simulink library "BEML_EMU_PantographInput_Lib"  (R2019b)
settings: Solver=VariableStepAuto  StartTime=0.0  StopTime=10.0  RelTol=1e-3
undefined symbols (not defined in the file): Control, Electrical, Environment, LineVoltage, NeutralSection, OverheadLinePresent, PantoADDFault, PantoControlPower, PantoDownCommand, PantographSampleTime, PantoIsolationCommand, PantoLoweringFailure, PantoMotorPower, PantoORDFault, PantoRaiseFailure, PantoUpCommand, Pneumatics
settings Model: Creator=rleighton  LastModifiedBy=hinganes
settings DataIOCC: ReturnWorkspaceOutputs=off
settings DebuggingCC: ArithmeticOperatorsInVariantConditions=warning
settings SFSimCC: SimUseLocalCustomCode=off  CustomCodeUndefinedFunction=UseInterfaceOnly
settings RTWCC: RTWUseLocalCustomCode=off

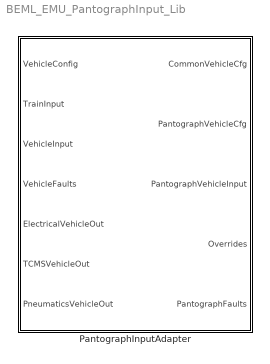
== system BEML_EMU_PantographInput_Lib ==
  PantographInputAdapter : Subsystem  TreatAsAtomicUnit=on  SystemSampleTime=PantographSampleTime

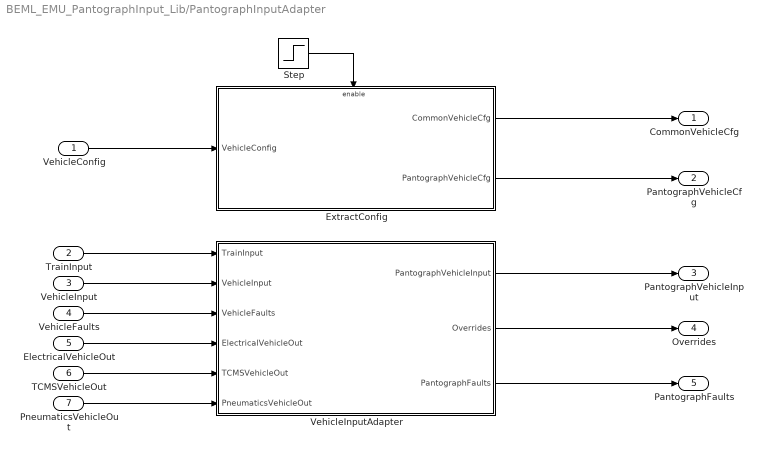
== system BEML_EMU_PantographInput_Lib/PantographInputAdapter ==
  VehicleConfig : Inport
  TrainInput : Inport  Port=2
  VehicleInput : Inport  Port=3
  VehicleFaults : Inport  Port=4
  ElectricalVehicleOut : Inport  Port=5
  TCMSVehicleOut : Inport  Port=6
  PneumaticsVehicleOut : Inport  Port=7
  ExtractConfig : Subsystem
  Step : Step  Before=1  After=0
  VehicleInputAdapter : Subsystem
  CommonVehicleCfg : Outport  VectorParamsAs1DForOutWhenUnconnected=off
  PantographVehicleCfg : Outport  Port=2  VectorParamsAs1DForOutWhenUnconnected=off
  PantographVehicleInput : Outport  Port=3  VectorParamsAs1DForOutWhenUnconnected=off
  Overrides : Outport  Port=4  VectorParamsAs1DForOutWhenUnconnected=off
  PantographFaults : Outport  Port=5  VectorParamsAs1DForOutWhenUnconnected=off
  wires:
  TrainInput/1 -> VehicleInputAdapter/1(TrainInput)
  VehicleInput/1 -> VehicleInputAdapter/2(VehicleInput)
  ElectricalVehicleOut/1 -> VehicleInputAdapter/4(ElectricalVehicleOut)
  PneumaticsVehicleOut/1 -> VehicleInputAdapter/6(PneumaticsVehicleOut)
  VehicleConfig/1 -> ExtractConfig/1(VehicleConfig)
  ExtractConfig/1(CommonVehicleCfg) -> CommonVehicleCfg/1
  ExtractConfig/2(PantographVehicleCfg) -> PantographVehicleCfg/1
  Step/1 -> ExtractConfig/Enable
  VehicleFaults/1 -> VehicleInputAdapter/3(VehicleFaults)
  VehicleInputAdapter/1(PantographVehicleInput) -> PantographVehicleInput/1
  VehicleInputAdapter/2(Overrides) -> Overrides/1
  VehicleInputAdapter/3(PantographFaults) -> PantographFaults/1
  TCMSVehicleOut/1 -> VehicleInputAdapter/5(TCMSVehicleOut)

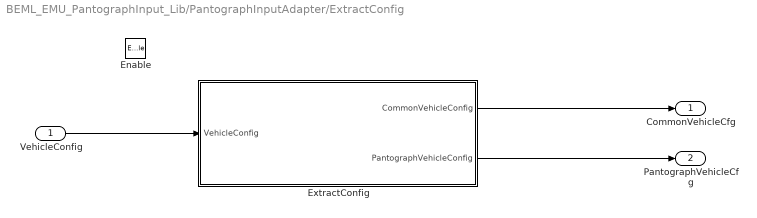
== system BEML_EMU_PantographInput_Lib/PantographInputAdapter/ExtractConfig ==
  VehicleConfig : Inport
  Enable : EnablePort
  ExtractConfig : Subsystem
  CommonVehicleCfg : Outport  VectorParamsAs1DForOutWhenUnconnected=off
  PantographVehicleCfg : Outport  Port=2  VectorParamsAs1DForOutWhenUnconnected=off
  wires:
  ExtractConfig/2(PantographVehicleConfig) -> PantographVehicleCfg/1
  ExtractConfig/1(CommonVehicleConfig) -> CommonVehicleCfg/1
  VehicleConfig/1 -> ExtractConfig/1(VehicleConfig)

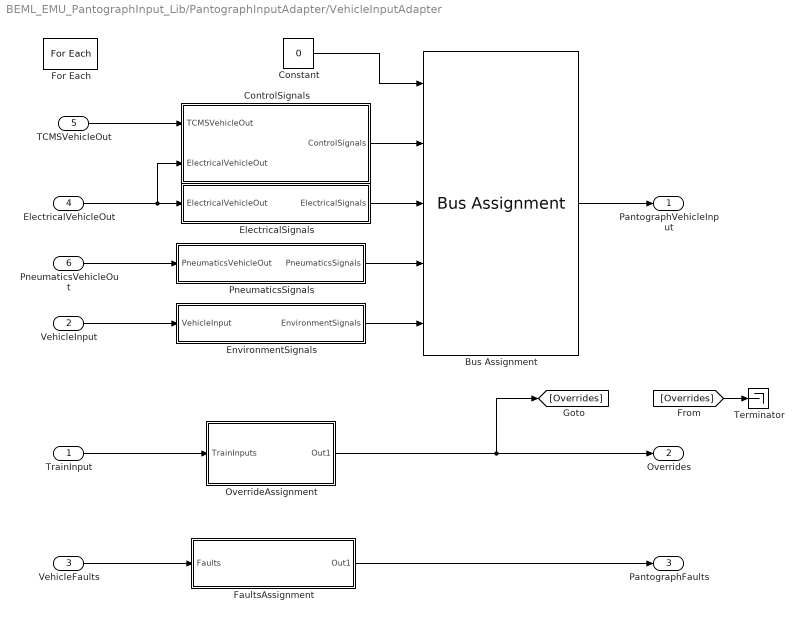
== system BEML_EMU_PantographInput_Lib/PantographInputAdapter/VehicleInputAdapter ==
  TrainInput : Inport
  VehicleInput : Inport  Port=2  Partition=on  PartitionDimension=1  PartitionWidth=1  PartitionOffset=0
  VehicleFaults : Inport  Port=3  Partition=on  PartitionDimension=1  PartitionWidth=1  PartitionOffset=0
  ElectricalVehicleOut : Inport  Port=4  Partition=on  PartitionDimension=1  PartitionWidth=1  PartitionOffset=0
  TCMSVehicleOut : Inport  Port=5  Partition=on  PartitionDimension=1  PartitionWidth=1  PartitionOffset=0
  PneumaticsVehicleOut : Inport  Port=6  Partition=on  PartitionDimension=1  PartitionWidth=1  PartitionOffset=0
  Bus Assignment : BusAssignment  AssignedSignals=Control,Electrical,Pneumatics,Environment
  Constant : Constant  Value=0  OutDataTypeStr=Bus: BD_PantographSystem_In_Vehicle
  ControlSignals : Subsystem
  ElectricalSignals : Subsystem
  EnvironmentSignals : Subsystem
  FaultsAssignment : Subsystem
  For Each : ForEach  DisableCoverage=on
  OverrideAssignment : Subsystem
  PneumaticsSignals : Subsystem
  Terminator : Terminator
  PantographVehicleInput : Outport  ConcatenationDimension=1  VectorParamsAs1DForOutWhenUnconnected=off
  Overrides : Outport  Port=2  ConcatenationDimension=1  VectorParamsAs1DForOutWhenUnconnected=off
  PantographFaults : Outport  Port=3  ConcatenationDimension=1  VectorParamsAs1DForOutWhenUnconnected=off
  wires:
  FaultsAssignment/1(Out1) -> PantographFaults/1
  VehicleFaults/1 -> FaultsAssignment/1(Faults)
  [Overrides] -> Terminator/1
  OverrideAssignment/1(Out1) -> [Overrides], Overrides/1
  TrainInput/1 -> OverrideAssignment/1(TrainInputs)
  EnvironmentSignals/1(EnvironmentSignals) -> Bus Assignment/5
  PneumaticsSignals/1(PneumaticsSignals) -> Bus Assignment/4
  VehicleInput/1 -> EnvironmentSignals/1(VehicleInput)
  ElectricalVehicleOut/1 -> ElectricalSignals/1(ElectricalVehicleOut), ControlSignals/2(ElectricalVehicleOut)
  Constant/1 -> Bus Assignment/1
  Bus Assignment/1 -> PantographVehicleInput/1
  ElectricalSignals/1(ElectricalSignals) -> Bus Assignment/3
  ControlSignals/1(ControlSignals) -> Bus Assignment/2
  PneumaticsVehicleOut/1 -> PneumaticsSignals/1(PneumaticsVehicleOut)
  TCMSVehicleOut/1 -> ControlSignals/1(TCMSVehicleOut)

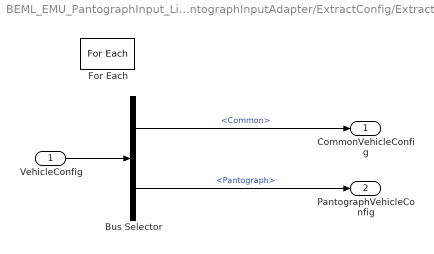
== system BEML_EMU_PantographInput_Lib/PantographInputAdapter/ExtractConfig/ExtractConfig ==
  VehicleConfig : Inport  Partition=on  PartitionDimension=1  PartitionWidth=1  PartitionOffset=0  BusOutputAsStruct=on
  Bus Selector : BusSelector  OutputSignals=Common,Pantograph
  For Each : ForEach  DisableCoverage=on
  CommonVehicleConfig : Outport  ConcatenationDimension=1  VectorParamsAs1DForOutWhenUnconnected=off
  PantographVehicleConfig : Outport  Port=2  ConcatenationDimension=1  VectorParamsAs1DForOutWhenUnconnected=off
  wires:
  VehicleConfig/1 -> Bus Selector/1
  Bus Selector/1 -> CommonVehicleConfig/1  "<Common>"
  Bus Selector/2 -> PantographVehicleConfig/1  "<Pantograph>"

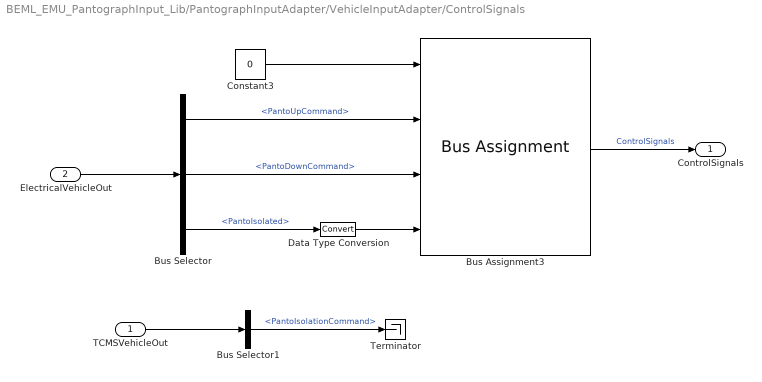
== system BEML_EMU_PantographInput_Lib/PantographInputAdapter/VehicleInputAdapter/ControlSignals ==
  TCMSVehicleOut : Inport
  ElectricalVehicleOut : Inport  Port=2
  Bus Assignment3 : BusAssignment  AssignedSignals=PantoUpCommand,PantoDownCommand,PantoIsolationCommand
  Bus Selector : BusSelector  OutputSignals=Pantograph.PantoUpCommand,Pantograph.PantoDownCommand,TCMS.PantoIsolated
  Bus Selector1 : BusSelector  OutputSignals=Control.PantographSystem.PantoIsolationCommand
  Constant3 : Constant  Value=0  OutDataTypeStr=Bus: BD_PantographSystem_In_Vehicle_Control
  Data Type Conversion : DataTypeConversion
  Terminator : Terminator
  ControlSignals : Outport
  wires:
  Data Type Conversion/1 -> Bus Assignment3/4
  Bus Selector/3 -> Data Type Conversion/1  "<PantoIsolated>"
  Bus Selector/2 -> Bus Assignment3/3  "<PantoDownCommand>"
  TCMSVehicleOut/1 -> Bus Selector1/1
  Bus Selector1/1 -> Terminator/1  "<PantoIsolationCommand>"
  ElectricalVehicleOut/1 -> Bus Selector/1
  Bus Assignment3/1 -> ControlSignals/1  "ControlSignals"
  Constant3/1 -> Bus Assignment3/1
  Bus Selector/1 -> Bus Assignment3/2  "<PantoUpCommand>"

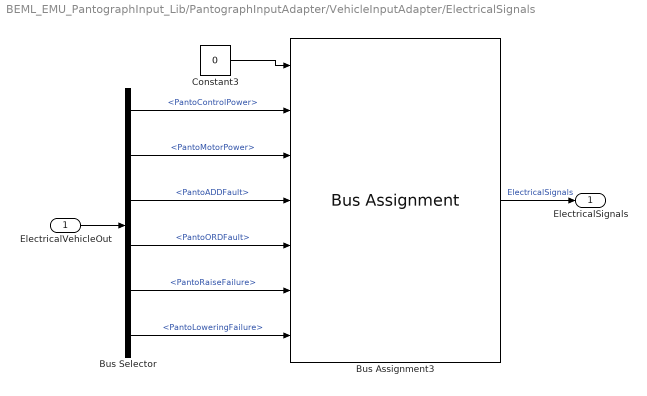
== system BEML_EMU_PantographInput_Lib/PantographInputAdapter/VehicleInputAdapter/ElectricalSignals ==
  ElectricalVehicleOut : Inport
  Bus Assignment3 : BusAssignment  AssignedSignals=PantoControlPower,PantoMotorPower,PantoADDFault,PantoORDFault,PantoRaiseFailure,PantoLoweringFailure
  Bus Selector : BusSelector  OutputSignals=Pantograph.PantoControlPower,Pantograph.PantoMotorPower,Pantograph.PantoADDFault,Pantograph.PantoORDFault,Pantograph.PantoRaiseFailure,Pantograph.PantoLoweringFailure
  Constant3 : Constant  Value=0  OutDataTypeStr=Bus: BD_PantographSystem_In_Vehicle_Electrical
  ElectricalSignals : Outport
  wires:
  Bus Selector/6 -> Bus Assignment3/7  "<PantoLoweringFailure>"
  Bus Selector/5 -> Bus Assignment3/6  "<PantoRaiseFailure>"
  Bus Selector/4 -> Bus Assignment3/5  "<PantoORDFault>"
  Bus Selector/3 -> Bus Assignment3/4  "<PantoADDFault>"
  ElectricalVehicleOut/1 -> Bus Selector/1
  Bus Assignment3/1 -> ElectricalSignals/1  "ElectricalSignals"
  Constant3/1 -> Bus Assignment3/1
  Bus Selector/1 -> Bus Assignment3/2  "<PantoControlPower>"
  Bus Selector/2 -> Bus Assignment3/3  "<PantoMotorPower>"

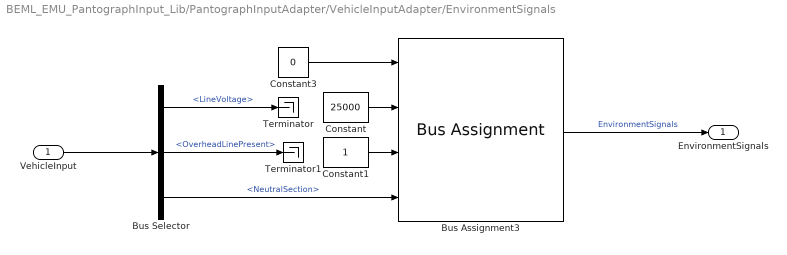
== system BEML_EMU_PantographInput_Lib/PantographInputAdapter/VehicleInputAdapter/EnvironmentSignals ==
  VehicleInput : Inport
  Bus Assignment3 : BusAssignment  AssignedSignals=LineVoltage,OverheadLinePresent,NeutralSection
  Bus Selector : BusSelector  OutputSignals=Environment.LineVoltage,Environment.OverheadLinePresent,Environment.NeutralSection
  Constant : Constant  Value=25000
  Constant1 : Constant
  Constant3 : Constant  Value=0  OutDataTypeStr=Bus: BD_PantographSystem_In_Vehicle_Environment
  Terminator : Terminator
  Terminator1 : Terminator
  EnvironmentSignals : Outport
  wires:
  Constant/1 -> Bus Assignment3/2
  Constant1/1 -> Bus Assignment3/3
  Bus Selector/3 -> Bus Assignment3/4  "<NeutralSection>"
  Bus Selector/2 -> Terminator1/1  "<OverheadLinePresent>"
  Bus Selector/1 -> Terminator/1  "<LineVoltage>"
  VehicleInput/1 -> Bus Selector/1
  Bus Assignment3/1 -> EnvironmentSignals/1  "EnvironmentSignals"
  Constant3/1 -> Bus Assignment3/1

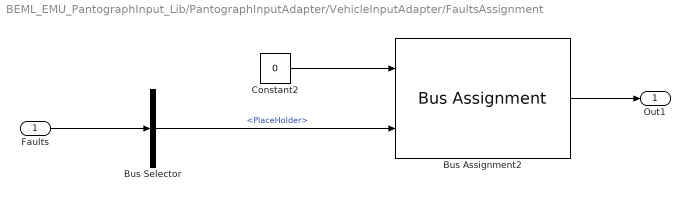
== system BEML_EMU_PantographInput_Lib/PantographInputAdapter/VehicleInputAdapter/FaultsAssignment ==
  Faults : Inport
  Bus Assignment2 : BusAssignment  AssignedSignals=PlaceHolder
  Bus Selector : BusSelector  OutputSignals=PantographFaults.PlaceHolder
  Constant2 : Constant  Value=0  OutDataTypeStr=Bus: BD_PantographSystem_In_Vehicle_Faults
  Out1 : Outport
  wires:
  Constant2/1 -> Bus Assignment2/1
  Bus Assignment2/1 -> Out1/1
  Faults/1 -> Bus Selector/1
  Bus Selector/1 -> Bus Assignment2/2  "<PlaceHolder>"

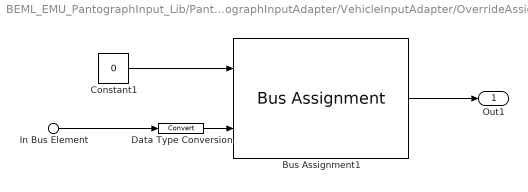
== system BEML_EMU_PantographInput_Lib/PantographInputAdapter/VehicleInputAdapter/OverrideAssignment ==
  In Bus Element : Inport  PortName=TrainInputs  Element=Overrides.AutoPowerOn
  Bus Assignment1 : BusAssignment  AssignedSignals=PantoUPOverride
  Constant1 : Constant  Value=0  OutDataTypeStr=Bus: BD_PantographSystem_In_Vehicle_Overrides
  Data Type Conversion : DataTypeConversion
  Out1 : Outport
  wires:
  In Bus Element/1 -> Data Type Conversion/1
  Data Type Conversion/1 -> Bus Assignment1/2
  Bus Assignment1/1 -> Out1/1
  Constant1/1 -> Bus Assignment1/1

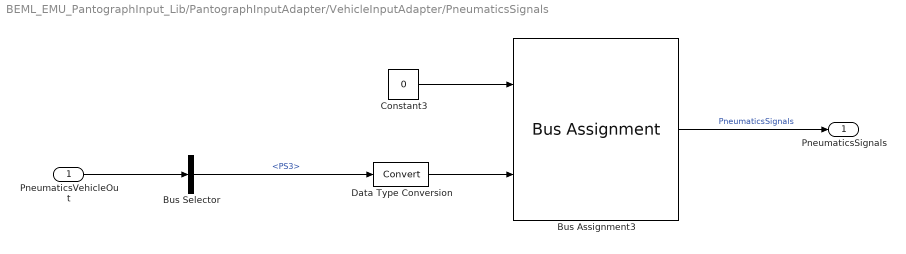
== system BEML_EMU_PantographInput_Lib/PantographInputAdapter/VehicleInputAdapter/PneumaticsSignals ==
  PneumaticsVehicleOut : Inport
  Bus Assignment3 : BusAssignment  AssignedSignals=PantoPneumaticSupply
  Bus Selector : BusSelector  OutputSignals=PressureSwitches.PS3
  Constant3 : Constant  Value=0  OutDataTypeStr=Bus: BD_PantographSystem_In_Vehicle_Pneumatics
  Data Type Conversion : DataTypeConversion
  PneumaticsSignals : Outport
  wires:
  Data Type Conversion/1 -> Bus Assignment3/2
  Bus Selector/1 -> Data Type Conversion/1  "<PS3>"
  Constant3/1 -> Bus Assignment3/1
  Bus Assignment3/1 -> PneumaticsSignals/1  "PneumaticsSignals"
  PneumaticsVehicleOut/1 -> Bus Selector/1
